simulink model "BLDCSpeedControl"  (R2020a)
settings: Solver=VariableStepAuto  StartTime=0.0  StopTime=10.0  RelTol=1e-3
undefined symbols (not defined in the file): Kd, Ki, Kp, Ts
libraries: powerlib x6, simulink x6
settings Model: Creator=Admin  LastModifiedBy=Admin

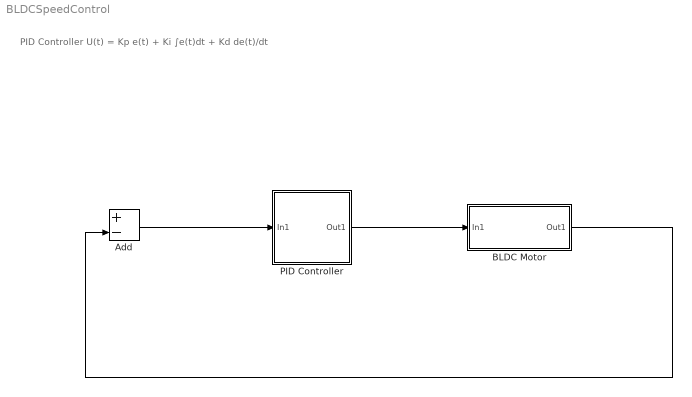
== system BLDCSpeedControl ==
  note: PID Controller
      |
      | U(t) = Kp e(t) + Ki ∫e(t)dt + Kd de(t)/dt
  Add : Sum  Inputs=+-
  BLDC Motor : Subsystem
  PID Controller : Subsystem
  wires:
  Add/1 -> PID Controller/1(In1)
  PID Controller/1(Out1) -> BLDC Motor/1(In1)
  ? -> Add/1
  BLDC Motor/1(Out1) -> Add/2

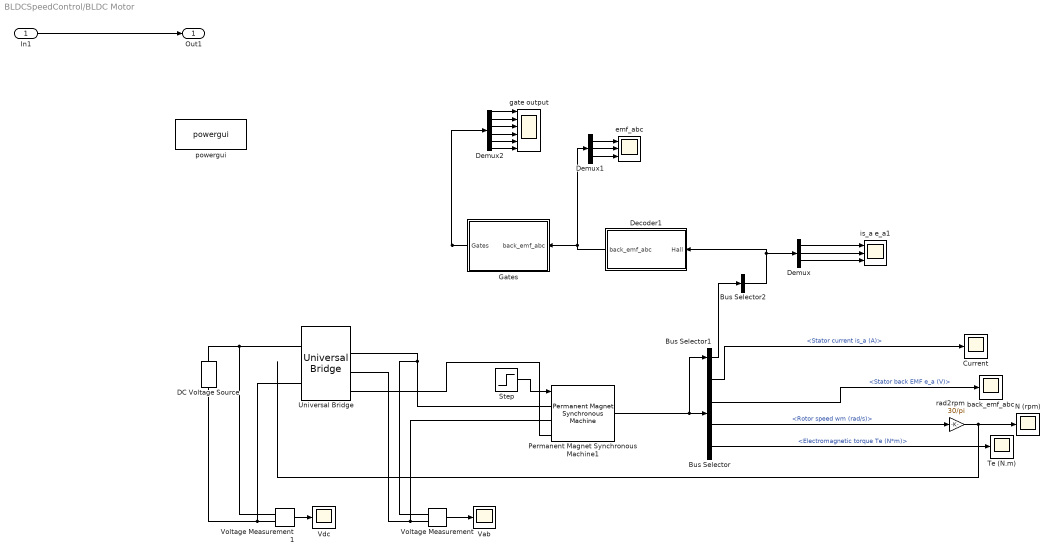
== system BLDCSpeedControl/BLDC Motor ==
  In1 : Inport
  Bus Selector : BusSelector  OutputSignals=Stator current is_a (A),Stator back EMF e_a (V),Rotor speed wm (rad/s),Electromagnetic torque Te (N*m)
  Bus Selector1 : BusSelector  OutputSignals=Hall effect signal h_a,Hall effect signal h_b,Hall effect signal h_c  OutputAsBus=on
  Bus Selector2 : BusSelector  OutputSignals=Hall effect signal h_a,Hall effect signal h_b,Hall effect signal h_c  OutputAsBus=on
  Current : Scope
  DC Voltage Source : powerlib/Electrical Sources/DC Voltage Source  Amplitude=300  Measurements=None
  Decoder1 : Subsystem
  Demux : Demux  Outputs=3
  Demux1 : Demux  Outputs=3
  Demux2 : Demux  Outputs=6
  Gates : Subsystem
  N (rpm) : Scope
  Permanent Magnet Synchronous Machine1 : powerlib/Machines/Permanent Magnet Synchronous Machine  NbPhases=3  FluxDistribution=Trapezoidal  RotorType=Round  MechanicalLoad=Torque Tm  PresetModel=No  ShowDetailedParameters=on  MeasurementBus=off  Resistance=2.8750  Inductance=8.5e-3  dqInductances=[8.5e-3, 8.5e-3]  La=0.000835  MachineConstant=Flux linkage established by magnets (V.s)  Flux=0.175  VoltageCst=146.6077  TorqueCst=1.4  Flat=120  Mechanical=[ 0.8e-3, 1e-3 4]  PolePairs=4  InitialConditions=[0,0, 0,0]  InitialConditions5ph=[0 0 0 0 0 0]  RefAngle=90 degrees behind phase A axis (modified Park)  IterativeDiscreteModel=Trapezoidal non iterative  TsBlock=-1  TsPowergui=0
  Step : Step  Time=.1  After=3  SampleTime=0
  Te (N.m) : Scope
  Universal Bridge : powerlib/Power Electronics/Universal Bridge  Arms=3  SnubberResistance=5000  SnubberCapacitance=1e-6  Device=MOSFET / Diodes  Ron=1e-3  Lon=0  ForwardVoltages="[  0  0  ]"  ForwardVoltage=0  GTOparameters=[ 10e-6 , 20e-6 ]  IGBTparameters=[ 1e-6 , 2e-6 ]  Measurements=None  Measurements_2=None  converterType=Rectifier
  Vab : Scope
  Vdc : Scope
  Voltage Measurement : powerlib/Measurements/Voltage Measurement  PhasorSimulation=off  OutputType=Complex  PSBequivalent=0
  Voltage Measurement1 : powerlib/Measurements/Voltage Measurement  PhasorSimulation=off  OutputType=Complex  PSBequivalent=0
  back_emf_abc : Scope
  emf_abc : Scope  NumInputPorts=3
  gate output : Scope  NumInputPorts=6
  is_a e_a1 : Scope  NumInputPorts=3
  powergui : powerlib/powergui  Priority=2  SimulationMode=Continuous  SampleTime=Ts  frequency=60  Iterations=50  frequencyindice=0  Pbase=100e6  ErrMax=1e-4  UnitsV=kV  UnitsW=MW  buscounter=0  FunctionMessages=off  echomessages=off  EnableUseOfTLC=off  CurrentSourceSwitches=off  DisableSnubberDevices=off  DisableRonSwitches=off  DisableVfSwitches=off  DisplayEquations=off  AutomaticDiscreteSolvers=off  SolverType=Tustin  Interpol=off  ExternalGateDelay=off  methode=off  Ts=0  x0status=blocks  SPID=off  SwTol=0  HookPort=off  NonlinearTolerance=1e-4  nMaxIteration=100  ContinueOnMaxIteration=off  RestoreLinks=warning  ResistiveCurrentMeasurement=off  Frange=[0:2:500]  Ylog=off  Xlog=on  ShowGrid=off  save=off  variable=ZData  structure=0  ZoomFFT=on  StartTime=0.0  cycles=1  DisplayStyle=1  fundamental=60  FreqAxis=off  MaxFrequency=1000  frequencyindicesteady=1  RmsSteady=1  display=off
  rad2rpm : Gain  Gain=30/pi
  Out1 : Outport
  wires:
  In1/1 -> Out1/1
  Voltage Measurement1/1 -> Vdc/1
  Voltage Measurement/1 -> Vab/1
  Demux2/6 -> gate output/6
  Gates/1(Gates) -> Demux2/1
  Demux2/4 -> gate output/4
  Demux2/2 -> gate output/2
  Demux2/1 -> gate output/1
  Demux2/5 -> gate output/5
  Demux2/3 -> gate output/3
  Decoder1/1(back_emf_abc) -> Demux1/1, Gates/1("back_emf_abc ")
  Demux1/2 -> emf_abc/2
  Demux1/3 -> emf_abc/3
  Demux1/1 -> emf_abc/1
  Step/1 -> Permanent Magnet Synchronous Machine1/1
  Bus Selector/1 -> Current/1  "<Stator current is_a (A)>"
  Bus Selector/2 -> back_emf_abc/1  "<Stator back EMF e_a (V)>"
  Bus Selector/3 -> rad2rpm/1  "<Rotor speed wm (rad/s)>"
  rad2rpm/1 -> N (rpm)/1
  Bus Selector/4 -> Te (N.m)/1  "<Electromagnetic torque Te (N*m)>"
  Permanent Magnet Synchronous Machine1/1 -> Bus Selector/1, Bus Selector1/1
  Demux/3 -> is_a e_a1/3
  Demux/2 -> is_a e_a1/2
  Demux/1 -> is_a e_a1/1
  Bus Selector2/1 -> Decoder1/1("Hall "), Demux/1
  Bus Selector1/1 -> Bus Selector2/1
  connections:
  DC Voltage Source/RConn1 -- Universal Bridge/RConn1 -- Voltage Measurement1/LConn1
  Voltage Measurement1/LConn2 -- DC Voltage Source/LConn1 -- Universal Bridge/RConn2
  Voltage Measurement/LConn2 -- Permanent Magnet Synchronous Machine1/LConn2 -- Universal Bridge/LConn2
  Voltage Measurement/LConn1 -- Permanent Magnet Synchronous Machine1/LConn1 -- Universal Bridge/LConn1
  Universal Bridge/LConn3 -- Permanent Magnet Synchronous Machine1/LConn3

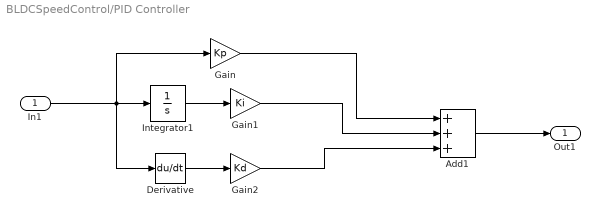
== system BLDCSpeedControl/PID Controller ==
  In1 : Inport
  Add1 : Sum  Inputs=+++
  Derivative : Derivative
  Gain : Gain  Gain=Kp
  Gain1 : Gain  Gain=Ki
  Gain2 : Gain  Gain=Kd
  Integrator1 : Integrator
  Out1 : Outport
  wires:
  Derivative/1 -> Gain2/1
  Integrator1/1 -> Gain1/1
  Gain1/1 -> Add1/2
  Add1/1 -> Out1/1
  Gain2/1 -> Add1/3
  In1/1 -> Derivative/1, Gain/1, Integrator1/1
  Gain/1 -> Add1/1

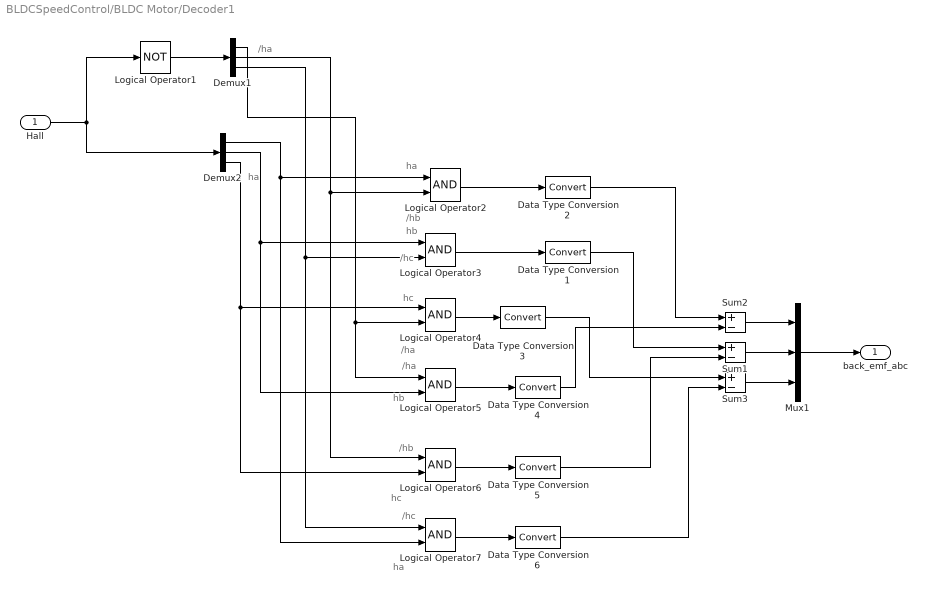
== system BLDCSpeedControl/BLDC Motor/Decoder1 ==
  note: /ha
  note: ha
  note: ha
  note: /hb
  note: hb
  note: /hc
  note: hc
  note: /ha
  note: /ha
  note: hb
  note: /hb
  note: hc
  note: /hc
  note: ha
  "Hall " : Inport
  Data Type Conversion{1..6} (6 alike) : DataTypeConversion
  Demux1 : Demux  Outputs=3
  Demux2 : Demux  Outputs=3
  Logical Operator1 : Logic  Operator=NOT  AllPortsSameDT=off  OutDataTypeStr=boolean
  Logical Operator{2..7} (6 alike) : Logic  AllPortsSameDT=off  OutDataTypeStr=boolean
  Mux1 : Mux  Inputs=3
  Sum1 : Sum  Inputs=+-  OutDataTypeStr=double
  Sum2 : Sum  Inputs=+-  OutDataTypeStr=double
  Sum3 : Sum  Inputs=+-  OutDataTypeStr=double
  back_emf_abc : Outport
  wires:
  "Hall "/1 -> Logical Operator1/1, Demux2/1
  Logical Operator1/1 -> Demux1/1
  Demux2/3 -> Logical Operator4/1, Logical Operator6/2
  Demux2/2 -> Logical Operator3/1, Logical Operator5/2
  Demux2/1 -> Logical Operator2/1, Logical Operator7/2
  Demux1/3 -> Logical Operator3/2, Logical Operator7/1
  Demux1/2 -> Logical Operator2/2, Logical Operator6/1
  Demux1/1 -> Logical Operator4/2, Logical Operator5/1
  Logical Operator2/1 -> Data Type Conversion2/1
  Sum2/1 -> Mux1/1
  Sum1/1 -> Mux1/2
  Sum3/1 -> Mux1/3
  Mux1/1 -> back_emf_abc/1
  Logical Operator3/1 -> Data Type Conversion1/1
  Logical Operator4/1 -> Data Type Conversion3/1
  Logical Operator5/1 -> Data Type Conversion4/1
  Logical Operator6/1 -> Data Type Conversion5/1
  Logical Operator7/1 -> Data Type Conversion6/1
  Data Type Conversion2/1 -> Sum2/1
  Data Type Conversion4/1 -> Sum2/2
  Data Type Conversion1/1 -> Sum1/1
  Data Type Conversion5/1 -> Sum1/2
  Data Type Conversion3/1 -> Sum3/1
  Data Type Conversion6/1 -> Sum3/2

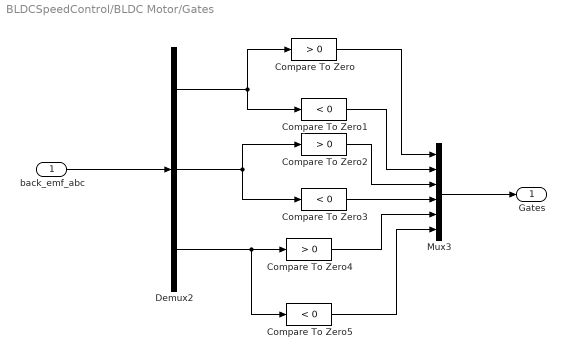
== system BLDCSpeedControl/BLDC Motor/Gates ==
  "back_emf_abc " : Inport
  Compare To Zero : simulink/Logic and Bit Operations/Compare To Zero  relop=>  OutDataTypeStr=boolean  ZeroCross=off
  Compare To Zero1 : simulink/Logic and Bit Operations/Compare To Zero  relop=<  OutDataTypeStr=boolean  ZeroCross=off
  Compare To Zero2 : simulink/Logic and Bit Operations/Compare To Zero  relop=>  OutDataTypeStr=boolean  ZeroCross=off
  Compare To Zero3 : simulink/Logic and Bit Operations/Compare To Zero  relop=<  OutDataTypeStr=boolean  ZeroCross=off
  Compare To Zero4 : simulink/Logic and Bit Operations/Compare To Zero  relop=>  OutDataTypeStr=boolean  ZeroCross=off
  Compare To Zero5 : simulink/Logic and Bit Operations/Compare To Zero  relop=<  OutDataTypeStr=boolean  ZeroCross=off
  Demux2 : Demux  Outputs=3
  Mux3 : Mux  Inputs=6
  Gates : Outport
  wires:
  "back_emf_abc "/1 -> Demux2/1
  Mux3/1 -> Gates/1
  Demux2/1 -> Compare To Zero/1, Compare To Zero1/1
  Demux2/2 -> Compare To Zero2/1, Compare To Zero3/1
  Demux2/3 -> Compare To Zero4/1, Compare To Zero5/1
  Compare To Zero/1 -> Mux3/1
  Compare To Zero1/1 -> Mux3/2
  Compare To Zero2/1 -> Mux3/3
  Compare To Zero3/1 -> Mux3/4
  Compare To Zero4/1 -> Mux3/5
  Compare To Zero5/1 -> Mux3/6
